simulink model "IEEE_1547_UI_TEST"  (R2018b)
settings: Solver=ode4  StartTime=0.0  StopTime=inf  FixedStep=Ts  RelTol=1e-3  EnableMultiTasking=on
PostLoadFcn:
  | Ts=40e-6; ARTEMIS_DISABLE_RTLAB_COMPATIBILTY_CHECK=1;
InitFcn:
  | Ts=40e-6; ARTEMIS_DISABLE_RTLAB_COMPATIBILTY_CHECK=1;
undefined symbols (not defined in the file or in its folder): another_event_name, I, Left, my_event_name, Right, type, V
libraries: simulink x72, powerlib_meascontrol x70, powerlib x66, artemis x4, rtlab x3, rtio_opalrt_ml605ex1 x3
(part 2 of 3)

== system IEEE_1547_UI_TEST/SC_InputsandOutputs/Subsystem9/Subsystem6 ==
  Inverter Measurements : Inport
  Bus Selector : BusSelector  OutputSignals=Inv VLL,Inv I,Inv Ptot pu,Inv Qtot pu,Inv Freq,Inv Pgen,Inv QFactor,Inv Ptot,Inv Qtot
  To Workspace : ToWorkspace  VariableName=Inv_VLL  SaveFormat=Timeseries  SampleTime=-1
  To Workspace1 : ToWorkspace  VariableName=Inv_I  SaveFormat=Timeseries  SampleTime=-1
  To Workspace2 : ToWorkspace  VariableName=Inv_Ptot_pu  SaveFormat=Timeseries  SampleTime=-1
  To Workspace3 : ToWorkspace  VariableName=Inv_Qtot_pu  SaveFormat=Timeseries  SampleTime=-1
  To Workspace4 : ToWorkspace  VariableName=Inv_Freq  SaveFormat=Timeseries  SampleTime=-1
  To Workspace5 : ToWorkspace  VariableName=Inv_Pgen  SaveFormat=Timeseries  SampleTime=-1
  To Workspace6 : ToWorkspace  VariableName=Inv_QFactor  SaveFormat=Timeseries  SampleTime=-1
  To Workspace7 : ToWorkspace  VariableName=Inv_Ptot  SaveFormat=Timeseries  SampleTime=-1
  To Workspace8 : ToWorkspace  VariableName=Inv_Qtot  SaveFormat=Timeseries  SampleTime=-1
  wires:
  Inverter Measurements/1 -> Bus Selector/1
  Bus Selector/1 -> To Workspace/1  "<Inv VLL>"
  Bus Selector/2 -> To Workspace1/1  "<Inv I>"
  Bus Selector/3 -> To Workspace2/1  "<Inv Ptot pu>"
  Bus Selector/4 -> To Workspace3/1  "<Inv Qtot pu>"
  Bus Selector/5 -> To Workspace4/1  "<Inv Freq>"
  Bus Selector/6 -> To Workspace5/1  "<Inv Pgen>"
  Bus Selector/7 -> To Workspace6/1  "<Inv QFactor>"
  Bus Selector/8 -> To Workspace7/1  "<Inv Ptot>"
  Bus Selector/9 -> To Workspace8/1  "<Inv Qtot>"

== system IEEE_1547_UI_TEST/SC_InputsandOutputs/Subsystem9/Subsystem7 ==
  Load Measurements : Inport
  Bus Selector : BusSelector  OutputSignals=Load Vph,Load Vll,Load I,Load Ppu,Load Qpu,Load PF,IR,IL,IC,PR pu,PL pu,QL pu,QC pu
  To Workspace1 : ToWorkspace  VariableName=Load_VLL  SaveFormat=Timeseries  SampleTime=-1
  To Workspace10 : ToWorkspace  VariableName=QL_pu  SaveFormat=Timeseries  SampleTime=-1
  To Workspace11 : ToWorkspace  VariableName=PL_pu  SaveFormat=Timeseries  SampleTime=-1
  To Workspace12 : ToWorkspace  VariableName=I_Capacitor  SaveFormat=Timeseries  SampleTime=-1
  To Workspace13 : ToWorkspace  VariableName=QC_PU  SaveFormat=Timeseries  SampleTime=-1
  To Workspace2 : ToWorkspace  VariableName=Load_Ptot_pu  SaveFormat=Timeseries  SampleTime=-1
  To Workspace3 : ToWorkspace  VariableName=Load_I  SaveFormat=Timeseries  SampleTime=-1
  To Workspace4 : ToWorkspace  VariableName=Load_PF  SaveFormat=Timeseries  SampleTime=-1
  To Workspace5 : ToWorkspace  VariableName=I_Inductor  SaveFormat=Timeseries  SampleTime=-1
  To Workspace6 : ToWorkspace  VariableName=I_Resistor  SaveFormat=Timeseries  SampleTime=-1
  To Workspace7 : ToWorkspace  VariableName=Load_Vph  SaveFormat=Timeseries  SampleTime=-1
  To Workspace8 : ToWorkspace  VariableName=Load_Qtot_pu  SaveFormat=Timeseries  SampleTime=-1
  To Workspace9 : ToWorkspace  VariableName=PR_pu  SaveFormat=Timeseries  SampleTime=-1
  wires:
  Load Measurements/1 -> Bus Selector/1
  Bus Selector/1 -> To Workspace7/1  "<Load Vph>"
  Bus Selector/2 -> To Workspace1/1  "<Load Vll>"
  Bus Selector/3 -> To Workspace3/1  "<Load I>"
  Bus Selector/4 -> To Workspace2/1  "<Load Ppu>"
  Bus Selector/5 -> To Workspace8/1  "<Load Qpu>"
  Bus Selector/6 -> To Workspace4/1  "<Load PF>"
  Bus Selector/7 -> To Workspace6/1  "<IR>"
  Bus Selector/8 -> To Workspace5/1  "<IL>"
  Bus Selector/9 -> To Workspace12/1  "<IC>"
  Bus Selector/10 -> To Workspace9/1  "<PR pu>"
  Bus Selector/11 -> To Workspace11/1  "<PL pu>"
  Bus Selector/12 -> To Workspace10/1  "<QL pu>"
  Bus Selector/13 -> To Workspace13/1  "<QC pu>"

== system IEEE_1547_UI_TEST/SC_InputsandOutputs/Subsystem9/Subsystem8 ==
  RLC Display Values : Inport
  Bus Selector : BusSelector  OutputSignals=Resistor (ohms),Rint (ohms),Inductor (mH),Capacitor (uF)
  To Workspace1 : ToWorkspace  VariableName=ohms_in_Rint  SaveFormat=Timeseries  SampleTime=-1
  To Workspace10 : ToWorkspace  VariableName=ohms_in_R  SaveFormat=Timeseries  SampleTime=-1
  To Workspace2 : ToWorkspace  VariableName=uF_in_C  SaveFormat=Timeseries  SampleTime=-1
  To Workspace3 : ToWorkspace  VariableName=mH_in_L  SaveFormat=Timeseries  SampleTime=-1
  wires:
  RLC Display Values/1 -> Bus Selector/1
  Bus Selector/1 -> To Workspace10/1  "<Resistor (ohms)>"
  Bus Selector/2 -> To Workspace1/1  "<Rint (ohms)>"
  Bus Selector/3 -> To Workspace3/1  "<Inductor (mH)>"
  Bus Selector/4 -> To Workspace2/1  "<Capacitor (uF)>"

== system IEEE_1547_UI_TEST/SM_SystemDynamics/ 3Phase Y Load with N/   C Bank ==
  note: Compensator for fixed time steps of 40e-6
  uC. : Inport
  AVG( RMS )1 : Subsystem
      mask Display: color('blue');disp('RMS\nAVG')
  Add1 : Sum  Inputs=2
  C1 : Subsystem
  C2 : Subsystem
  C3 : Subsystem
  Divide : Product
  Mux : Mux  Inputs=3
  Mux1 : Mux  Inputs=3
  Opposite of P_L : Constant  Value=-1
  Power per Element : Subsystem
      mask Display:
      | color('red')
      | disp('Power          \nper               \nElement       ')
  "Power, 3Ph (  Fund. Frecu. )" : Subsystem
  A : PMIOPort  Side=Left
  B : PMIOPort  Port=2  Side=Left
  C : PMIOPort  Port=3  Side=Left
  a : PMIOPort  Port=4  Side=Right
  b : PMIOPort  Port=5  Side=Right
  c : PMIOPort  Port=6  Side=Right
  P_VC : Outport
  Q_C : Outport  Port=2
  tag scope: I_C=global, P_C=global
  wires:
  uC./1 -> C1/1(uC), C3/1(uC), C2/1(uC)
  "Power, 3Ph (  Fund. Frecu. )"/2(Q) -> Q_C/1
  "Power, 3Ph (  Fund. Frecu. )"/1(P) -> [P_C]
  C2/1(V_C) -> Mux/3
  C3/2(I_C) -> Mux1/1
  C1/2(I_C) -> Mux1/2
  C3/1(V_C) -> Mux/1
  C1/1(V_C) -> Mux/2
  C2/2(I_C) -> Mux1/3
  Add1/1 -> P_VC/1
  [P_C] -> Divide/1, Add1/1
  Divide/1 -> Add1/2
  Opposite of P_L/1 -> Divide/2
  AVG( RMS )1/1(Out1) -> [I_C]
  Mux/1 -> Power per Element/1(Vabc), "Power, 3Ph (  Fund. Frecu. )"/1(Vabc)
  Mux1/1 -> Power per Element/2(Iabc), "Power, 3Ph (  Fund. Frecu. )"/2(Iabc), AVG( RMS )1/1(In1)
  connections:
  C3/RConn2 -- a/RConn1
  C1/RConn1 -- B/RConn1
  C3/RConn1 -- A/RConn1
  C2/RConn2 -- c/RConn1
  C1/RConn2 -- b/RConn1
  C2/RConn1 -- C/RConn1

== system IEEE_1547_UI_TEST/SM_SystemDynamics/ 3Phase Y Load with N/   R Bank1 ==
  ohms : Inport
  "3Ph ( P.U. ) Power, Fund. Frec." : Subsystem
  AVG( RMS )4 : Subsystem
      mask Display: color('blue');disp('RMS\nAVG')
  Mux : Mux  Inputs=3
  Mux1 : Mux  Inputs=3
  Power per Element : Subsystem
      mask Display:
      | color('red')
      | disp('Power          \nper               \nElement       ')
  R1 : Subsystem
  R2 : Subsystem
  R3 : Subsystem
  A : PMIOPort  Side=Left
  B : PMIOPort  Port=2  Side=Left
  C : PMIOPort  Port=3  Side=Left
  a : PMIOPort  Port=4  Side=Right
  b : PMIOPort  Port=5  Side=Right
  c : PMIOPort  Port=6  Side=Right
  P_RL : Outport
  Q_RL : Outport  Port=2
  tag scope: I_R=global
  wires:
  R1/1(V) -> Mux/1
  R2/2(I) -> Mux1/2
  R3/2(I) -> Mux1/3
  R1/2(I) -> Mux1/1
  R2/1(V) -> Mux/2
  R3/1(V) -> Mux/3
  "3Ph ( P.U. ) Power, Fund. Frec."/1(P) -> P_RL/1
  "3Ph ( P.U. ) Power, Fund. Frec."/2(Q) -> Q_RL/1
  ohms/1 -> R1/1(ohms), R3/1(ohms), R2/1(ohms)
  AVG( RMS )4/1(Out1) -> [I_R]
  Mux1/1 -> AVG( RMS )4/1(In1), Power per Element/2(Iabc), "3Ph ( P.U. ) Power, Fund. Frec."/2(Iabc)
  Mux/1 -> Power per Element/1(Vabc), "3Ph ( P.U. ) Power, Fund. Frec."/1(Vabc)
  connections:
  R2/RConn2 -- b/RConn1
  R3/RConn2 -- c/RConn1
  R1/RConn2 -- a/RConn1
  R1/RConn1 -- A/RConn1
  R2/RConn1 -- B/RConn1
  R3/RConn1 -- C/RConn1

== system IEEE_1547_UI_TEST/SM_SystemDynamics/ 3Phase Y Load with N/( Rint + L ) Bank ==
  mH : Inport
  Rint : Inport  Port=2
  AVG( RMS )1 : Subsystem
      mask Display: color('blue');disp('RMS\nAVG')
  Add : Sum  Inputs=2
  L1 : Subsystem
  L2 : Subsystem
  L3 : Subsystem
  Mean2 : powerlib_meascontrol/Measurements/Mean  Freq=30  Vinit=0  Ts=Ts
      settings: SourceProductName=Simscape Electrical
  Mux2 : Mux  Inputs=3
  Mux3 : Mux  Inputs=3
  Power per Element : Subsystem
      mask Display:
      | color('red')
      | disp('Power          \nper               \nElement       ')
  "Power, 3Ph (  Fund. Frecu. )" : Subsystem
  A : PMIOPort  Side=Left
  B : PMIOPort  Port=2  Side=Left
  C : PMIOPort  Port=3  Side=Left
  a : PMIOPort  Port=4  Side=Right
  b : PMIOPort  Port=5  Side=Right
  c : PMIOPort  Port=6  Side=Right
  P_L : Outport
  Q_L : Outport  Port=2
  tag scope: I_L=global
  wires:
  L1/2(I_L) -> Mux3/1
  L2/2(I_L) -> Mux3/2
  L3/2(I_L) -> Mux3/3
  mH/1 -> L3/1(mH), L2/1(mH), L1/1(mH)
  Rint/1 -> L3/2(Rint), L2/2(Rint), L1/2(Rint)
  L2/1(V_L) -> Mux2/2
  L3/1(V_L) -> Mux2/3
  "Power, 3Ph (  Fund. Frecu. )"/2(Q) -> Q_L/1
  L1/1(V_L) -> Mux2/1
  [P_C] -> Add/1
  "Power, 3Ph (  Fund. Frecu. )"/1(P) -> Add/2
  Add/1 -> Mean2/1
  AVG( RMS )1/1(Out1) -> [I_L]
  Mean2/1 -> P_L/1
  Mux2/1 -> Power per Element/1(Vabc), "Power, 3Ph (  Fund. Frecu. )"/1(Vabc)
  Mux3/1 -> Power per Element/2(Iabc), AVG( RMS )1/1(In1), "Power, 3Ph (  Fund. Frecu. )"/2(Iabc)
  connections:
  L1/RConn2 -- a/RConn1
  L2/RConn2 -- b/RConn1
  L3/RConn2 -- c/RConn1
  L3/RConn1 -- C/RConn1
  L1/RConn1 -- A/RConn1
  L2/RConn1 -- B/RConn1

== system IEEE_1547_UI_TEST/SM_SystemDynamics/Inverter Measurements/AVG( RMS )2 ==
  In1 : Inport
  Mean : powerlib_meascontrol/Measurements/Mean  Freq=60  Vinit=0  Ts=0
      settings: SourceProductName=Simscape Electrical
  RMS : powerlib_meascontrol/Measurements/RMS  TrueRMS=on  Freq=60  RMSInit=120  Ts=Ts
      settings: SourceProductName=Simscape Electrical
  Out1 : Outport
  wires:
  Mean/1 -> Out1/1
  RMS/1 -> Mean/1
  In1/1 -> RMS/1

== system IEEE_1547_UI_TEST/SM_SystemDynamics/Inverter Measurements/AVG( RMS )6 ==
  In1 : Inport
  Mean : powerlib_meascontrol/Measurements/Mean  Freq=60  Vinit=0  Ts=Ts
      settings: SourceProductName=Simscape Electrical
  RMS : powerlib_meascontrol/Measurements/RMS  TrueRMS=on  Freq=60  RMSInit=120  Ts=Ts
      settings: SourceProductName=Simscape Electrical
  Out1 : Outport
  wires:
  Mean/1 -> Out1/1
  RMS/1 -> Mean/1
  In1/1 -> RMS/1

== system IEEE_1547_UI_TEST/SM_SystemDynamics/Inverter Measurements/Inverter Performance ==
  P_inv_pu : Inport
  P_Load_pu : Inport  Port=2
  Q_inv_pu : Inport  Port=3
  Q_L_pu : Inport  Port=4
  Q_C_pu : Inport  Port=5
  Abs : Abs
  Abs1 : Abs
  Add : Sum
  Add1 : Sum
  Compare To Constant1 : simulink/Logic and Bit Operations/Compare To Constant  relop=<  const=0  OutDataTypeStr=boolean
  Compare To Constant3 : simulink/Logic and Bit Operations/Compare To Constant  relop=>  const=0  OutDataTypeStr=boolean
  Divide : Product  Inputs=*/  SaturateOnIntegerOverflow=on  RndMeth=Zero
  Divide1 : Product  Inputs=**  SaturateOnIntegerOverflow=on  RndMeth=Zero
  Divide2 : Product  Inputs=**  SaturateOnIntegerOverflow=on  RndMeth=Zero
  Divide3 : Product  Inputs=**  SaturateOnIntegerOverflow=on  RndMeth=Zero
  Divide4 : Product  Inputs=/*  SaturateOnIntegerOverflow=on  RndMeth=Zero
  Divide5 : Product  Inputs=*/  SaturateOnIntegerOverflow=on  RndMeth=Zero
  Divide6 : Product  Commented=on  Inputs=**  SaturateOnIntegerOverflow=on  RndMeth=Zero
  Divide8 : Product  Commented=on  Inputs=**  SaturateOnIntegerOverflow=on  RndMeth=Zero
  Saturation : Saturate  Commented=through  UpperLimit=inf  LowerLimit=0.0001
  Saturation1 : Saturate  Commented=through  UpperLimit=inf  LowerLimit=0.0001
  Sqrt : Sqrt  SaturateOnIntegerOverflow=on
  Sqrt1 : Sqrt  Commented=on  SaturateOnIntegerOverflow=on
  Sqrt2 : Sqrt  Commented=on  SaturateOnIntegerOverflow=on
  P Gen : Outport
  Q factor : Outport  Port=2
  wires:
  P_inv_pu/1 -> Divide/1
  Compare To Constant3/1 -> Divide1/1
  Compare To Constant1/1 -> Divide2/2
  Q_inv_pu/1 -> Compare To Constant1/1, Compare To Constant3/1, Abs/1
  Divide1/1 -> Add/2
  Abs/1 -> Divide1/2, Divide2/1
  Q_L_pu/1 -> Add/1
  Divide2/1 -> Add1/1
  Q_C_pu/1 -> Abs1/1
  Add/1 -> Divide3/1, Divide5/1
  Divide3/1 -> Sqrt/1
  Sqrt/1 -> Divide4/2
  Divide4/1 -> Q factor/1
  Abs1/1 -> Add1/2
  Divide5/1 -> Sqrt1/1
  Sqrt1/1 -> Divide6/1
  Divide6/1 -> ?  "Freq_Island"
  ? -> Divide6/2  "Freq_EPS"
  Divide/1 -> Sqrt2/1, P Gen/1
  Sqrt2/1 -> Divide8/2
  ? -> Divide8/1  "Vph_Uti"
  Divide8/1 -> ?  "V_Island"
  P_Load_pu/1 -> Saturation1/1
  Add1/1 -> Saturation/1, Divide3/2
  Saturation/1 -> Divide5/2
  Saturation1/1 -> Divide/2, Divide4/1

== system IEEE_1547_UI_TEST/SM_SystemDynamics/Inverter Measurements/Phase Angle Meter1 ==
  Vabc : Inport
  Iabc : Inport  Port=2
  Constant : Constant  Value=-1
  Cos : Trigonometry  Operator=cos
  Gain : Gain  Gain=pi/180
  PLL (3ph) : powerlib_meascontrol/PLL/PLL (3ph)  Fmin=30  Par_Init=[0, 60]  ParK=[180, 3200, 1]  TcD=1e-4  MaxRateChangeFreq=12  FilterCutOffFreq=25  Ts=Ts  AGC=on
  Positive-Sequence (PLL-Driven) : powerlib_meascontrol/Measurements/Positive-Sequence (PLL-Driven)  Finit=60  Fmin=45  InInit=[1, 0]  Ts=Ts
      settings: SourceProductName=Simscape Power Systems  SourceProductBaseCode=PS
  Product : Product  Inputs=3
  Sign : Signum
  Θ : Outport
  pf : Outport  Port=2
  wires:
  PLL (3ph)/1 -> Positive-Sequence (PLL-Driven)/1
  PLL (3ph)/2 -> Positive-Sequence (PLL-Driven)/2
  Iabc/1 -> Positive-Sequence (PLL-Driven)/3
  Vabc/1 -> PLL (3ph)/1
  Positive-Sequence (PLL-Driven)/2 -> Gain/1, Sign/1, Θ/1
  Product/1 -> pf/1
  Gain/1 -> Cos/1
  Cos/1 -> Product/3
  Constant/1 -> Product/2
  Sign/1 -> Product/1

== system IEEE_1547_UI_TEST/SM_SystemDynamics/Inverter Measurements/Power, 3Ph ( Fundamental Frecuency ) ==
  note: Per Unit Converter
  note: Per Unit Converter
  Vabc : Inport
  Iabc : Inport  Port=2
  Inv Size : Inport  Port=3
  Divide : Product  Inputs=*/
  Divide1 : Product  Inputs=*/
  Gain : Gain
  Gain1 : Gain
  Mean1 : powerlib_meascontrol/Measurements/Mean  Freq=30  Vinit=0  Ts=Ts
      settings: SourceProductName=Simscape Electrical
  Mean2 : powerlib_meascontrol/Measurements/Mean  Freq=30  Vinit=0  Ts=Ts
      settings: SourceProductName=Simscape Electrical
  PLL (3ph) : powerlib_meascontrol/PLL/PLL (3ph)  Fmin=45  Par_Init=[0, 60]  ParK=[180, 3200, 1]  TcD=1e-4  MaxRateChangeFreq=12  FilterCutOffFreq=25  Ts=Ts  AGC=on
      settings: SourceProductName=Simscape Electrical
  Power ( Fundamental Frecuency ) : powerlib_meascontrol/Measurements/Power (PLL-Driven, Positive-Sequence)  Finit=60  Fmin=45  Vinit=[1, 0]  Iinit=[1, 0]  Ts=Ts
      settings: SourceProductName=Simscape Electrical  SourceProductBaseCode=PS
  P : Outport
  Ppu : Outport  Port=2
  Q : Outport  Port=3
  Qpu : Outport  Port=4
  Inv Freq : Outport  Port=5
  wires:
  Mean2/1 -> P/1, Divide/1
  Gain/1 -> Divide/2
  Power ( Fundamental Frecuency )/1 -> Mean2/1
  Mean1/1 -> Q/1, Divide1/1
  Gain1/1 -> Divide1/2
  Power ( Fundamental Frecuency )/2 -> Mean1/1
  Divide/1 -> Ppu/1
  Divide1/1 -> Qpu/1
  Inv Size/1 -> Gain/1, Gain1/1
  PLL (3ph)/1 -> Inv Freq/1, Power ( Fundamental Frecuency )/1
  PLL (3ph)/2 -> Power ( Fundamental Frecuency )/2
  Vabc/1 -> Power ( Fundamental Frecuency )/3, PLL (3ph)/1
  Iabc/1 -> Power ( Fundamental Frecuency )/4

== system IEEE_1547_UI_TEST/SM_SystemDynamics/MASTER CONTROL OUTPUTS/INVERTER MEASURES ==
  Bus Creator : BusCreator  Inputs=10
  Inv Freq : Gain
  Inv I : Gain
  Inv Pgen : Gain
  Inv Ptot : Gain
  Inv Ptot pu : Gain
  Inv Qfactor : Gain
  Inv Qtot : Gain
  Inv Qtot pu : Gain
  Inv Vph : Gain
  Inv Vph pu : Gain  Gain=1/277
  Subsystem : Subsystem
  Subsystem1 : Subsystem
  Inverter Measures : Outport
  wires:
  Subsystem/1(Out1) -> Inv Vph pu/1, Inv Vph/1  "Inv Vph"
  [Pinv_pu] -> Inv Ptot pu/1  "Inv Ptot pu"
  [Qinv_pu] -> Inv Qtot pu/1  "Inv Qtot pu"
  Subsystem1/1(Out1) -> Inv Freq/1  "Inv Freq"
  [p_gen] -> Inv Pgen/1  "Inv Pgen"
  [q_Factor] -> Inv Qfactor/1  "Inv QFactor"
  [P_inv] -> Inv Ptot/1  "Inv Ptot"
  [Q_inv] -> Inv Qtot/1  "Inv Qtot"
  [inv_I] -> Inv I/1  "Inv I"
  Bus Creator/1 -> Inverter Measures/1
  Inv I/1 -> Bus Creator/3  "Inv I"
  Inv Freq/1 -> Bus Creator/6  "Inv Freq"
  Inv Pgen/1 -> Bus Creator/7  "Inv Pgen"
  Inv Ptot/1 -> Bus Creator/9  "Inv Ptot"
  Inv Ptot pu/1 -> Bus Creator/4  "Inv Ptot pu"
  Inv Qfactor/1 -> Bus Creator/8  "Inv QFactor"
  Inv Qtot/1 -> Bus Creator/10  "Inv Qtot"
  Inv Qtot pu/1 -> Bus Creator/5  "Inv Qtot pu"
  Inv Vph/1 -> Bus Creator/1  "Inv Vph"
  Inv Vph pu/1 -> Bus Creator/2  "Inv Vph PU"
  [stop_ametek] -> Subsystem/1(trig)
  [inv_Vph] -> Subsystem/2(input)  "Inv Vph"
  [stop_ametek] -> Subsystem1/1(trig)
  [Inv_Freq] -> Subsystem1/2(input)  "Inv Freq"

== system IEEE_1547_UI_TEST/SM_SystemDynamics/MASTER CONTROL OUTPUTS/LOAD MEASURES ==
  Bus Creator : BusCreator  Inputs=15
  IC : Gain
  IL : Gain
  IR : Gain
  Load I : Gain
  Load PF : Gain
  Load Ppu : Gain
  Load Qpu : Gain
  Load Vph : Gain
  Load Vph pu : Gain  Gain=1/277
  PL pu : Gain
  PLoad Watts : Gain
  PR pu : Gain
  QC pu : Gain
  QL pu : Gain
  QLoad Vars : Gain
  Load Measures : Outport
  wires:
  [pf] -> Load PF/1  "Load PF"
  [load_Vph] -> Load Vph pu/1, Load Vph/1  "Load Vph"
  [load_I] -> Load I/1  "Load I"
  [PLpu] -> Load Ppu/1  "Load Ppu"
  [QLpu] -> Load Qpu/1  "Load Qpu"
  [I_R] -> IR/1  "IR"
  [I_L] -> IL/1  "IL"
  [I_C] -> IC/1  "IC"
  [P_RL] -> PR pu/1  "PR pu"
  [P_L] -> PL pu/1  "PL pu"
  [Q_L] -> QL pu/1  "QL pu"
  [Q_C] -> QC pu/1  "QC pu"
  Bus Creator/1 -> Load Measures/1
  Load Vph/1 -> Bus Creator/1  "Load Vph"
  Load Vph pu/1 -> Bus Creator/2  "Load Vph pu"
  Load I/1 -> Bus Creator/3  "Load I"
  Load Ppu/1 -> Bus Creator/4  "Load Ppu"
  Load Qpu/1 -> Bus Creator/5  "Load Qpu"
  Load PF/1 -> Bus Creator/6  "Load PF"
  IR/1 -> Bus Creator/7  "IR"
  IL/1 -> Bus Creator/8  "IL"
  IC/1 -> Bus Creator/9  "IC"
  PR pu/1 -> Bus Creator/10  "PR pu"
  PL pu/1 -> Bus Creator/11  "PL pu"
  QL pu/1 -> Bus Creator/12  "QL pu"
  QC pu/1 -> Bus Creator/13  "QC pu"
  QLoad Vars/1 -> Bus Creator/15  "QLoad Vars"
  PLoad Watts/1 -> Bus Creator/14  "PLoad Watts"
  [P_load_Watts] -> PLoad Watts/1
  [Q_load_Vars] -> QLoad Vars/1

== system IEEE_1547_UI_TEST/SM_SystemDynamics/MASTER CONTROL OUTPUTS/RLC DISPLAYED VALUES ==
  Bus Creator : BusCreator  Inputs=7
  C in uF : Gain
  FreqPCC : Gain
  L in mh : Gain
  R in ohms : Gain
  Rint in ohms : Gain
  Spare O1 : Gain
  Spare O2 : Gain
  RLC Displayed Values : Outport
  wires:
  [ohms7] -> Rint in ohms/1
  [ohms2] -> R in ohms/1
  [uF2] -> C in uF/1
  [mH2] -> L in mh/1
  Bus Creator/1 -> RLC Displayed Values/1
  C in uF/1 -> Bus Creator/4  "Capacitor (uF)"
  R in ohms/1 -> Bus Creator/1  "Resistor (ohms)"
  Rint in ohms/1 -> Bus Creator/2  "Rint (ohms)"
  L in mh/1 -> Bus Creator/3  "Inductor (mH)"
  FreqPCC/1 -> Bus Creator/5  "Freq PCC"
  [FreqPCC] -> FreqPCC/1
  Spare O2/1 -> Bus Creator/6  "Spare O2"
  [Spare_O2] -> Spare O2/1
  Spare O1/1 -> Bus Creator/7  "Spare O1"
  [Spare_O1] -> Spare O1/1

== system IEEE_1547_UI_TEST/SM_SystemDynamics/MASTER CONTROL OUTPUTS/SPARE MEASURES ==
  Bus Creator2 : BusCreator  Inputs=5
  Islanding Signal : Gain  Gain=-1
  OpMonitor : rtlab/Monitoring/OpMonitor  compute_time=off  real_step=off  idle_time=off  nb_overruns=on  user_time=off  user_name=my_event_name,another_event_name
      settings: SourceProductName=RT-LAB
  Phase Angle : Gain
  Spare O3 : Gain
  pf_inv : Gain
  Spare Measures : Outport
  wires:
  [Islanding_Test] -> Islanding Signal/1
  [pf_inv] -> pf_inv/1
  [Spare_O3] -> Spare O3/1
  [Phase_Angle] -> Phase Angle/1
  Bus Creator2/1 -> Spare Measures/1
  Islanding Signal/1 -> Bus Creator2/3  "Island Sig"
  Phase Angle/1 -> Bus Creator2/2  "Phase Angle"
  Spare O3/1 -> Bus Creator2/5  "Spare O3"
  pf_inv/1 -> Bus Creator2/1  "pf_inv"
  OpMonitor/1 -> Bus Creator2/4  "Overruns"

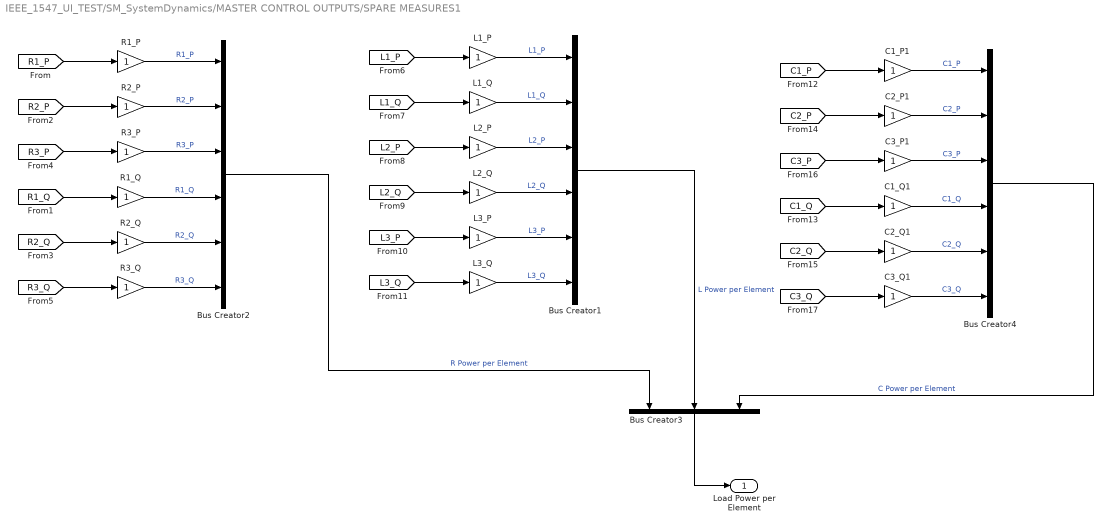
== system IEEE_1547_UI_TEST/SM_SystemDynamics/MASTER CONTROL OUTPUTS/SPARE MEASURES1 ==
  Bus Creator1 : BusCreator  Inputs=6
  Bus Creator2 : BusCreator  Inputs=6
  Bus Creator3 : BusCreator  Inputs=3
  Bus Creator4 : BusCreator  Inputs=6
  C1_P1 : Gain
  C1_Q1 : Gain
  C2_P1 : Gain
  C2_Q1 : Gain
  C3_P1 : Gain
  C3_Q1 : Gain
  L1_P : Gain
  L1_Q : Gain
  L2_P : Gain
  L2_Q : Gain
  L3_P : Gain
  L3_Q : Gain
  R1_P : Gain
  R1_Q : Gain
  R2_P : Gain
  R2_Q : Gain
  R3_P : Gain
  R3_Q : Gain
  Load Power per Element : Outport
  wires:
  R3_P/1 -> Bus Creator2/3  "R3_P"
  R2_P/1 -> Bus Creator2/2  "R2_P"
  R2_Q/1 -> Bus Creator2/5  "R2_Q"
  R1_P/1 -> Bus Creator2/1  "R1_P"
  R1_Q/1 -> Bus Creator2/4  "R1_Q"
  R3_Q/1 -> Bus Creator2/6  "R3_Q"
  [R1_P] -> R1_P/1
  [R1_Q] -> R1_Q/1
  [R2_P] -> R2_P/1
  [R3_P] -> R3_P/1
  [R2_Q] -> R2_Q/1
  [R3_Q] -> R3_Q/1
  Bus Creator1/1 -> Bus Creator3/2  "L Power per Element"
  L2_P/1 -> Bus Creator1/3  "L2_P"
  [L3_P] -> L3_P/1
  L3_P/1 -> Bus Creator1/5  "L3_P"
  [L3_Q] -> L3_Q/1
  [L1_Q] -> L1_Q/1
  [L1_P] -> L1_P/1
  L2_Q/1 -> Bus Creator1/4  "L2_Q"
  [L2_Q] -> L2_Q/1
  L1_P/1 -> Bus Creator1/1  "L1_P"
  L1_Q/1 -> Bus Creator1/2  "L1_Q"
  L3_Q/1 -> Bus Creator1/6  "L3_Q"
  [L2_P] -> L2_P/1
  Bus Creator3/1 -> Load Power per Element/1
  Bus Creator2/1 -> Bus Creator3/1  "R Power per Element"
  C2_P1/1 -> Bus Creator4/2  "C2_P"
  [C3_P] -> C3_P1/1
  C3_P1/1 -> Bus Creator4/3  "C3_P"
  [C3_Q] -> C3_Q1/1
  [C1_Q] -> C1_Q1/1
  [C1_P] -> C1_P1/1
  C2_Q1/1 -> Bus Creator4/5  "C2_Q"
  [C2_Q] -> C2_Q1/1
  C1_P1/1 -> Bus Creator4/1  "C1_P"
  C1_Q1/1 -> Bus Creator4/4  "C1_Q"
  C3_Q1/1 -> Bus Creator4/6  "C3_Q"
  [C2_P] -> C2_P1/1
  Bus Creator4/1 -> Bus Creator3/3  "C Power per Element"

== system IEEE_1547_UI_TEST/SM_SystemDynamics/MASTER CONTROL OUTPUTS/SPARE MEASURES2 ==
  Bus Creator2 : BusCreator  Inputs=12
  S1_P : Gain
  S1_P_Pu : Gain
  S1_Q : Gain
  S1_Q_Pu : Gain
  S2_P : Gain
  S2_P_Pu : Gain
  S2_Q : Gain
  S2_Q_Pu : Gain
  S3_P : Gain
  S3_P_Pu : Gain
  S3_Q : Gain
  S3_Q_Pu : Gain
  Switch Power : Outport
  wires:
  S3_P/1 -> Bus Creator2/3  "S3_P_Watts"
  S2_P/1 -> Bus Creator2/2  "S2_P_Watts"
  S2_Q/1 -> Bus Creator2/5  "S2_Q_Vars"
  S1_P/1 -> Bus Creator2/1  "S1_P_Watts"
  S1_Q/1 -> Bus Creator2/4  "S1_Q_Vars"
  S3_Q/1 -> Bus Creator2/6  "S3_Q_Vars"
  [S1_Watts] -> S1_P/1
  [S1_Vars] -> S1_Q/1
  [S2_Watts] -> S2_P/1
  [S3_Watts] -> S3_P/1
  Bus Creator2/1 -> Switch Power/1  "Switch Power"
  [S3_Vars] -> S3_Q/1
  [S2_Vars] -> S2_Q/1
  [S3_P_Pu] -> S3_P_Pu/1
  [S3_Q_Pu] -> S3_Q_Pu/1
  S3_P_Pu/1 -> Bus Creator2/9  "S3_P_Pu"
  S3_Q_Pu/1 -> Bus Creator2/12  "S3_Q_Pu"
  [S1_P_Pu] -> S1_P_Pu/1
  S1_P_Pu/1 -> Bus Creator2/7  "S1_P_Pu"
  S1_Q_Pu/1 -> Bus Creator2/10  "S1_Q_Pu"
  [S1_Q_Pu] -> S1_Q_Pu/1
  [S2_P_Pu] -> S2_P_Pu/1
  S2_P_Pu/1 -> Bus Creator2/8  "S2_P_Pu"
  [S2_Q_Pu] -> S2_Q_Pu/1
  S2_Q_Pu/1 -> Bus Creator2/11  "S2_Q_Pu"

== system IEEE_1547_UI_TEST/SM_SystemDynamics/MASTER CONTROL OUTPUTS/UTILITY MEASURES ==
  Bus Creator : BusCreator  Inputs=7
  PFun : Gain
  QFun : Gain
  Uti I : Gain
  Uti Ppu : Gain
  Uti Qpu : Gain
  Uti Vph : Gain
  Uti Vph pu : Gain  Gain=1/277
  Utility Measures : Outport
  wires:
  Bus Creator/1 -> Utility Measures/1
  [uti_I] -> Uti I/1  "Utility I"
  [Vph_Uti] -> Uti Vph pu/1, Uti Vph/1  "Utility Vph"
  [Puti_pu] -> Uti Ppu/1  "Utility Ppu"
  [Quti_pu] -> Uti Qpu/1  "Utility Qpu"
  [Puti_Watts] -> PFun/1
  [Quti_Vars] -> QFun/1
  Uti I/1 -> Bus Creator/3  "Utility I"
  Uti Vph/1 -> Bus Creator/1  "Utility Vph"
  Uti Qpu/1 -> Bus Creator/5  "Utility Qpu"
  Uti Ppu/1 -> Bus Creator/4  "Utility Ppu"
  Uti Vph pu/1 -> Bus Creator/2  "Utility Vph pu"
  PFun/1 -> Bus Creator/6  "Puti_Watts"
  QFun/1 -> Bus Creator/7  "Quti_Vars"

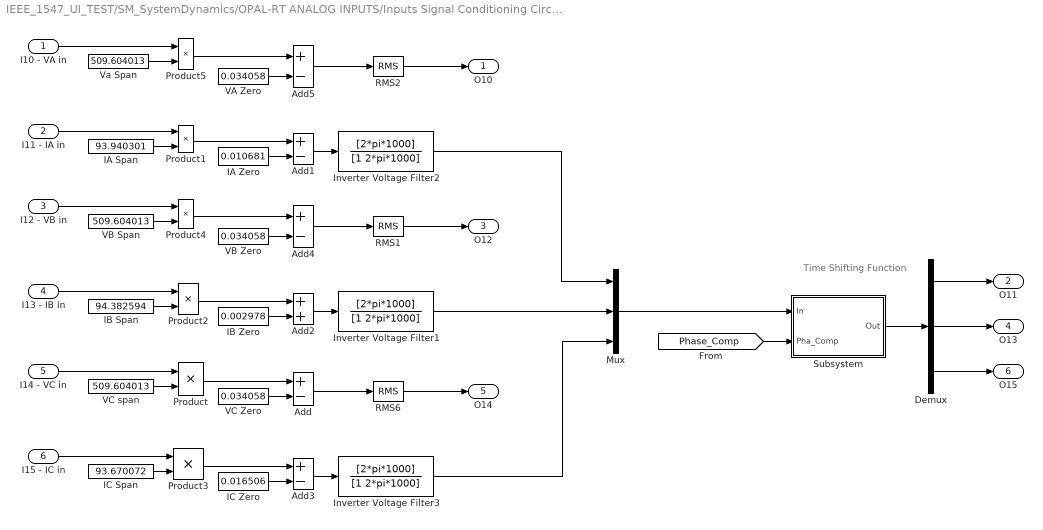
== system IEEE_1547_UI_TEST/SM_SystemDynamics/OPAL-RT ANALOG INPUTS/Inputs Signal Conditioning Circuit ==
  note: Time Shifting
      | Function
  I10 - VA in : Inport
  I11 - IA in : Inport  Port=2
  I12 - VB in : Inport  Port=3
  I13 - IB in : Inport  Port=4
  I14 - VC in : Inport  Port=5
  I15 - IC in : Inport  Port=6
  Add{,1,3..5} (5 alike) : Sum  Inputs=+-
  Add2 : Sum
  Demux : Demux  Outputs=3
  IA Span : Constant  Value=93.940301
  IA Zero : Constant  Value=0.010681
  IB Span : Constant  Value=94.382594
  IB Zero : Constant  Value=0.002978
  IC Span : Constant  Value=93.670072
  IC Zero : Constant  Value=0.016506
  Inverter Voltage Filter1 : TransferFcn  Numerator=[2*pi*1000]  Denominator=[1 2*pi*1000]
  Inverter Voltage Filter2 : TransferFcn  Numerator=[2*pi*1000]  Denominator=[1 2*pi*1000]
  Inverter Voltage Filter3 : TransferFcn  Numerator=[2*pi*1000]  Denominator=[1 2*pi*1000]
  Mux : Mux  Inputs=3
  Product{,1..5} (6 alike) : Product
  RMS1 : powerlib_meascontrol/Measurements/RMS  TrueRMS=on  Freq=60  RMSInit=120  Ts=0
      settings: SourceProductName=Simscape Electrical
  RMS2 : powerlib_meascontrol/Measurements/RMS  TrueRMS=on  Freq=60  RMSInit=120  Ts=0
      settings: SourceProductName=Simscape Electrical
  RMS6 : powerlib_meascontrol/Measurements/RMS  TrueRMS=on  Freq=60  RMSInit=120  Ts=0
      settings: SourceProductName=Simscape Electrical
  Subsystem : Subsystem
  VA Zero : Constant  Value=0.034058
  VB Span : Constant  Value=509.604013
  VB Zero : Constant  Value=0.034058
  VC Zero : Constant  Value=0.034058
  VC span : Constant  Value=509.604013
  Va Span : Constant  Value=509.604013
  "O10 " : Outport
  "O11 " : Outport  Port=2
  " O12" : Outport  Port=3
  " O13" : Outport  Port=4
  " O14" : Outport  Port=5
  " O15" : Outport  Port=6
  wires:
  RMS2/1 -> "O10 "/1
  IB Span/1 -> Product2/2
  VC span/1 -> Product/2
  IC Span/1 -> Product3/2
  VC Zero/1 -> Add/2
  Product/1 -> Add/1
  VB Span/1 -> Product4/2
  Add4/1 -> RMS1/1
  IB Zero/1 -> Add2/2
  IC Zero/1 -> Add3/2
  Product3/1 -> Add3/1
  Add1/1 -> Inverter Voltage Filter2/1
  Add2/1 -> Inverter Voltage Filter1/1
  Product2/1 -> Add2/1
  Add/1 -> RMS6/1
  IA Span/1 -> Product1/2
  Add3/1 -> Inverter Voltage Filter3/1
  Add5/1 -> RMS2/1
  Va Span/1 -> Product5/2
  I10 - VA in/1 -> Product5/1
  Inverter Voltage Filter3/1 -> Mux/3
  Inverter Voltage Filter2/1 -> Mux/1
  RMS1/1 -> " O12"/1
  I11 - IA in/1 -> Product1/1
  I12 - VB in/1 -> Product4/1
  I14 - VC in/1 -> Product/1
  I13 - IB in/1 -> Product2/1
  I15 - IC in/1 -> Product3/1
  RMS6/1 -> " O14"/1
  Inverter Voltage Filter1/1 -> Mux/2
  VB Zero/1 -> Add4/2
  Product4/1 -> Add4/1
  IA Zero/1 -> Add1/2
  Product1/1 -> Add1/1
  VA Zero/1 -> Add5/2
  Product5/1 -> Add5/1
  Mux/1 -> Subsystem/1(In)
  Subsystem/1(Out) -> Demux/1
  [Phase_Comp] -> Subsystem/2("Pha_Comp ")
  Demux/1 -> "O11 "/1
  Demux/2 -> " O13"/1
  Demux/3 -> " O15"/1

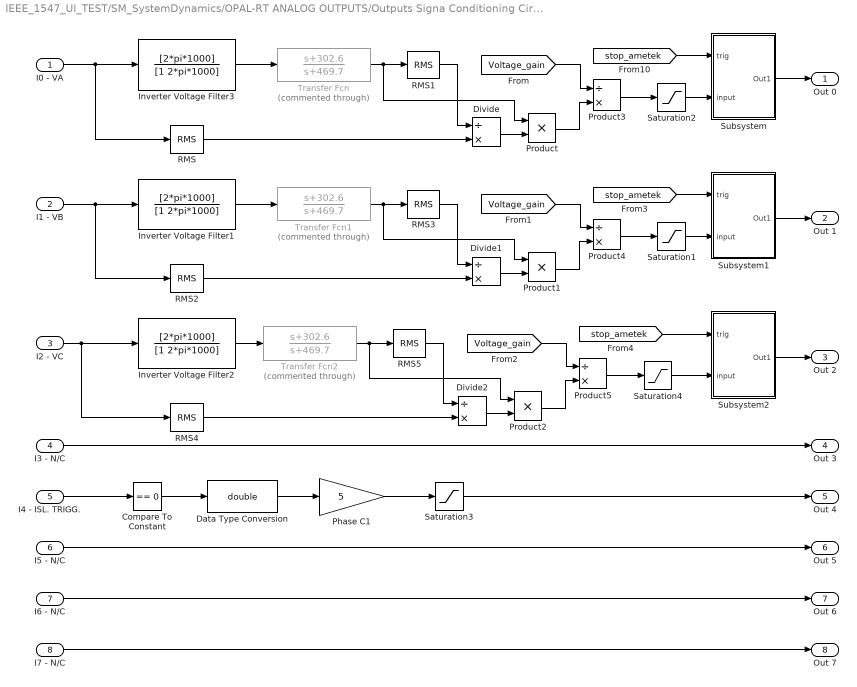
== system IEEE_1547_UI_TEST/SM_SystemDynamics/OPAL-RT ANALOG OUTPUTS/Outputs Signa Conditioning Circuit ==
  I0 - VA : Inport
  I1 - VB : Inport  Port=2
  I2 - VC : Inport  Port=3
  I3 - N/C : Inport  Port=4
  I4 - ISL. TRIGG. : Inport  Port=5
  I5 - N/C : Inport  Port=6
  I6 - N/C : Inport  Port=7
  I7 - N/C : Inport  Port=8
  Compare To Constant : simulink/Logic and Bit Operations/Compare To Constant  relop===  const=0  OutDataTypeStr=boolean
  Data Type Conversion : DataTypeConversion  OutDataTypeStr=double
  Divide : Product  Inputs=/*
  Divide1 : Product  Inputs=/*
  Divide2 : Product  Inputs=/*
  Inverter Voltage Filter1 : TransferFcn  Numerator=[2*pi*1000]  Denominator=[1 2*pi*1000]
  Inverter Voltage Filter2 : TransferFcn  Numerator=[2*pi*1000]  Denominator=[1 2*pi*1000]
  Inverter Voltage Filter3 : TransferFcn  Numerator=[2*pi*1000]  Denominator=[1 2*pi*1000]
  Phase C1 : Gain  Gain=5
  Product : Product
  Product1 : Product
  Product2 : Product
  Product3 : Product  Inputs=/*
  Product4 : Product  Inputs=/*
  Product5 : Product  Inputs=/*
  RMS{,1..5} (6 alike) : powerlib_meascontrol/Measurements/RMS  TrueRMS=on  Freq=60  RMSInit=120  Ts=Ts
      settings: SourceProductName=Simscape Electrical
  Saturation1 : Saturate  UpperLimit=10.2  LowerLimit=-10.2
  Saturation2 : Saturate  UpperLimit=10.2  LowerLimit=-10.2
  Saturation3 : Saturate  UpperLimit=5  LowerLimit=0
  Saturation4 : Saturate  UpperLimit=10.2  LowerLimit=-10.2
  Subsystem : Subsystem
  Subsystem1 : Subsystem
  Subsystem2 : Subsystem
  Transfer Fcn : TransferFcn  Commented=through  Numerator=[1 302.6]  Denominator=[1 469.7]
  Transfer Fcn1 : TransferFcn  Commented=through  Numerator=[1 302.6]  Denominator=[1 469.7]
  Transfer Fcn2 : TransferFcn  Commented=through  Numerator=[1 302.6]  Denominator=[1 469.7]
  Out 0 : Outport
  Out 1 : Outport  Port=2
  Out 2 : Outport  Port=3
  Out 3 : Outport  Port=4
  Out 4 : Outport  Port=5
  Out 5 : Outport  Port=6
  Out 6 : Outport  Port=7
  Out 7 : Outport  Port=8
  wires:
  I3 - N/C/1 -> Out 3/1
  I5 - N/C/1 -> Out 5/1
  I6 - N/C/1 -> Out 6/1
  I7 - N/C/1 -> Out 7/1
  I4 - ISL. TRIGG./1 -> Compare To Constant/1
  Saturation3/1 -> Out 4/1
  Compare To Constant/1 -> Data Type Conversion/1
  Data Type Conversion/1 -> Phase C1/1
  Inverter Voltage Filter3/1 -> Transfer Fcn/1
  I0 - VA/1 -> RMS/1, Inverter Voltage Filter3/1
  Transfer Fcn/1 -> Product/1, RMS1/1
  RMS/1 -> Divide/2
  RMS1/1 -> Divide/1
  Divide/1 -> Product/2
  Product3/1 -> Saturation2/1
  Saturation2/1 -> Subsystem/2(input)
  Phase C1/1 -> Saturation3/1
  Product/1 -> Product3/2
  [Voltage_gain] -> Product3/1
  Subsystem/1(Out1) -> Out 0/1
  [stop_ametek] -> Subsystem/1(trig)
  Product1/1 -> Product4/2
  Transfer Fcn1/1 -> Product1/1, RMS3/1
  RMS2/1 -> Divide1/2
  [Voltage_gain] -> Product4/1
  [stop_ametek] -> Subsystem1/1(trig)
  Product4/1 -> Saturation1/1
  Divide1/1 -> Product1/2
  Saturation1/1 -> Subsystem1/2(input)
  RMS3/1 -> Divide1/1
  Inverter Voltage Filter1/1 -> Transfer Fcn1/1
  I1 - VB/1 -> RMS2/1, Inverter Voltage Filter1/1
  Product2/1 -> Product5/2
  Transfer Fcn2/1 -> Product2/1, RMS5/1
  RMS4/1 -> Divide2/2
  [Voltage_gain] -> Product5/1
  [stop_ametek] -> Subsystem2/1(trig)
  Product5/1 -> Saturation4/1
  Divide2/1 -> Product2/2
  Saturation4/1 -> Subsystem2/2(input)
  RMS5/1 -> Divide2/1
  Inverter Voltage Filter2/1 -> Transfer Fcn2/1
  I2 - VC/1 -> RMS4/1, Inverter Voltage Filter2/1
  Subsystem1/1(Out1) -> Out 1/1
  Subsystem2/1(Out1) -> Out 2/1

== system IEEE_1547_UI_TEST/SM_SystemDynamics/PHIL SOFTWARE SIDE CURRENT SOURCES/Subsystem ==
  trig : Inport
  input : Inport  Port=2
  Constant : Constant  Value=0
  Switch : Switch  Criteria=u2 > Threshold
  Out1 : Outport
  wires:
  Switch/1 -> Out1/1
  trig/1 -> Switch/2
  Constant/1 -> Switch/3
  input/1 -> Switch/1

== system IEEE_1547_UI_TEST/SM_SystemDynamics/PHIL SOFTWARE SIDE CURRENT SOURCES/Subsystem1 ==
  trig : Inport
  input : Inport  Port=2
  Constant : Constant  Value=0
  Switch : Switch  Criteria=u2 > Threshold
  Out1 : Outport
  wires:
  Switch/1 -> Out1/1
  trig/1 -> Switch/2
  Constant/1 -> Switch/3
  input/1 -> Switch/1

== system IEEE_1547_UI_TEST/SM_SystemDynamics/PHIL SOFTWARE SIDE CURRENT SOURCES/Subsystem2 ==
  trig : Inport
  input : Inport  Port=2
  Constant : Constant  Value=0
  Switch : Switch  Criteria=u2 > Threshold
  Out1 : Outport
  wires:
  Switch/1 -> Out1/1
  trig/1 -> Switch/2
  Constant/1 -> Switch/3
  input/1 -> Switch/1

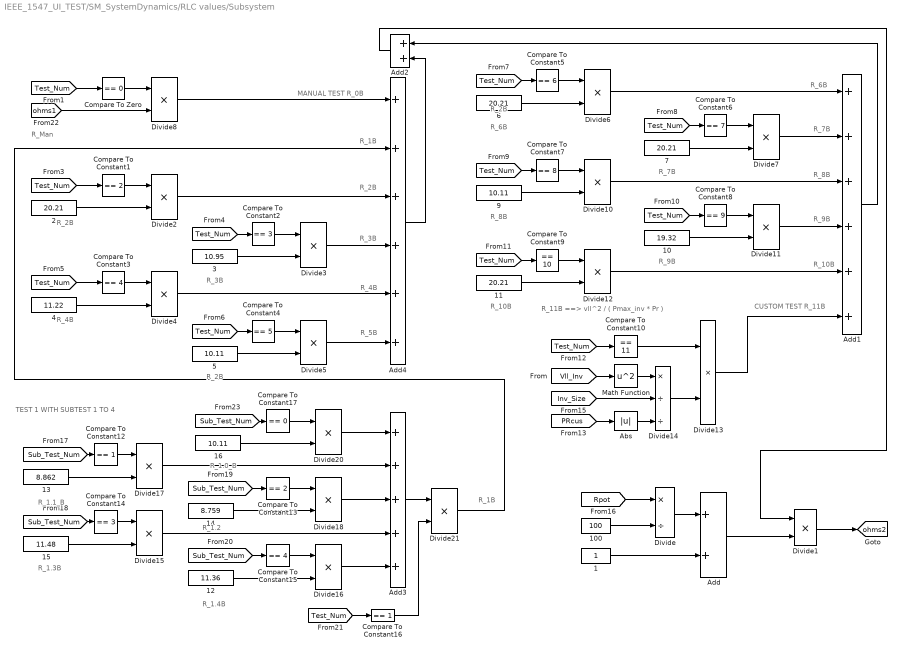
== system IEEE_1547_UI_TEST/SM_SystemDynamics/RLC values/Subsystem ==
  note: R_2B
  note: R_4B
  note: TEST 1 WITH SUBTEST 1 TO 4
  note: R_3B
  note: R_4B
  note: R_7B
  note: MANUAL TEST R_0B
  note: R_9B
  note: CUSTOM TEST R_11B
  note: R_5B
  note: R_Man
  note: R_11B ==> vll^2 / ( Pmax_inv * Pr )
  note: R_8B
  note: R_2B
  note: R_1.2
  note: R_10B
  note: R_6B
  note: R_2B
  note: R_1.3B
  note: R_10B
  note: R_9B
  note: R_8B
  note: R_1B
  note: R_1.0_B
  note: R_6B
  note: R_2B
  note: R_3B
  note: R_1.1_B
  note: R_1B
  note: R_1.4B
  note: R_7B
  1 : Constant
  10 : Constant  Value=19.32
  100 : Constant  Value=100
  {2,6..7,11} (4 alike) : Constant  Value=20.21
  12 : Constant  Value=11.36
  13 : Constant  Value=8.862
  14 : Constant  Value=8.759
  15 : Constant  Value=11.48
  16 : Constant  Value=10.11
  3 : Constant  Value=10.95
  4 : Constant  Value=11.22
  5 : Constant  Value=10.11
  9 : Constant  Value=10.11
  Abs : Abs
  Add : Sum
  Add1 : Sum  Inputs=++++++
  Add2 : Sum
  Add3 : Sum  Inputs=+++++
  Add4 : Sum  Inputs=++++++
  Compare To Constant1 : simulink/Logic and Bit Operations/Compare To Constant  relop===  const=2  OutDataTypeStr=boolean
  Compare To Constant10 : simulink/Logic and Bit Operations/Compare To Constant  relop===  const=11  OutDataTypeStr=boolean
  Compare To Constant12 : simulink/Logic and Bit Operations/Compare To Constant  relop===  const=1  OutDataTypeStr=boolean
  Compare To Constant13 : simulink/Logic and Bit Operations/Compare To Constant  relop===  const=2  OutDataTypeStr=boolean
  Compare To Constant14 : simulink/Logic and Bit Operations/Compare To Constant  relop===  const=3  OutDataTypeStr=boolean
  Compare To Constant15 : simulink/Logic and Bit Operations/Compare To Constant  relop===  const=4  OutDataTypeStr=boolean
  Compare To Constant16 : simulink/Logic and Bit Operations/Compare To Constant  relop===  const=1  OutDataTypeStr=boolean
  Compare To Constant17 : simulink/Logic and Bit Operations/Compare To Constant  relop===  const=0  OutDataTypeStr=boolean
  Compare To Constant2 : simulink/Logic and Bit Operations/Compare To Constant  relop===  const=3  OutDataTypeStr=boolean
  Compare To Constant3 : simulink/Logic and Bit Operations/Compare To Constant  relop===  const=4  OutDataTypeStr=boolean
  Compare To Constant4 : simulink/Logic and Bit Operations/Compare To Constant  relop===  const=5  OutDataTypeStr=boolean
  Compare To Constant5 : simulink/Logic and Bit Operations/Compare To Constant  relop===  const=6  OutDataTypeStr=boolean
  Compare To Constant6 : simulink/Logic and Bit Operations/Compare To Constant  relop===  const=7  OutDataTypeStr=boolean
  Compare To Constant7 : simulink/Logic and Bit Operations/Compare To Constant  relop===  const=8  OutDataTypeStr=boolean
  Compare To Constant8 : simulink/Logic and Bit Operations/Compare To Constant  relop===  const=9  OutDataTypeStr=boolean
  Compare To Constant9 : simulink/Logic and Bit Operations/Compare To Constant  relop===  const=10  OutDataTypeStr=boolean
  Compare To Zero : simulink/Logic and Bit Operations/Compare To Zero  relop===  OutDataTypeStr=boolean
  Divide : Product  Inputs=*/
  Divide{1..8,10..13,15..18,20..21} (18 alike) : Product  Inputs=**
  Divide14 : Product  Inputs=*//
  Math Function : Math  Operator=square  SaturateOnIntegerOverflow=on
  tag scope: ohms2=global
  wires:
  Divide1/1 -> [ohms2]
  Compare To Constant13/1 -> Divide18/1
  Add2/1 -> Divide1/1
  Add3/1 -> Divide21/1
  [Test_Num] -> Compare To Constant2/1
  Compare To Constant16/1 -> Divide21/2
  14/1 -> Divide18/2
  [Test_Num] -> Compare To Constant1/1
  Add/1 -> Divide1/2
  Divide13/1 -> Add1/6
  Divide20/1 -> Add3/1
  12/1 -> Divide16/2
  Compare To Constant17/1 -> Divide20/1
  [Sub_Test_Num] -> Compare To Constant17/1
  5/1 -> Divide5/2
  [Test_Num] -> Compare To Constant4/1
  Divide18/1 -> Add3/3
  Divide4/1 -> Add4/5
  Divide16/1 -> Add3/5
  Compare To Constant14/1 -> Divide15/1
  [Sub_Test_Num] -> Compare To Constant13/1
  7/1 -> Divide7/2
  [Sub_Test_Num] -> Compare To Constant12/1
  Compare To Constant2/1 -> Divide3/1
  [Test_Num] -> Compare To Constant16/1
  [Rpot] -> Divide/1
  Divide15/1 -> Add3/4
  Math Function/1 -> Divide14/1
  Divide8/1 -> Add4/1
  15/1 -> Divide15/2
  Compare To Constant15/1 -> Divide16/1
  [Sub_Test_Num] -> Compare To Constant14/1
  Compare To Constant9/1 -> Divide12/1
  Compare To Constant5/1 -> Divide6/1
  [Test_Num] -> Compare To Constant10/1
  Add4/1 -> Add2/2
  [Sub_Test_Num] -> Compare To Constant15/1
  Add1/1 -> Add2/1
  [Test_Num] -> Compare To Constant6/1
  Divide17/1 -> Add3/2
  [Test_Num] -> Compare To Constant8/1
  Compare To Constant6/1 -> Divide7/1
  Divide7/1 -> Add1/2
  [Inv_Size] -> Divide14/2
  9/1 -> Divide10/2
  Divide11/1 -> Add1/4
  Divide14/1 -> Divide13/2
  Compare To Constant8/1 -> Divide11/1
  Divide10/1 -> Add1/3
  [Vll_Inv] -> Math Function/1
  11/1 -> Divide12/2
  Compare To Zero/1 -> Divide8/1
  [Test_Num] -> Compare To Constant5/1
  Compare To Constant10/1 -> Divide13/1
  [Test_Num] -> Compare To Constant7/1
  Compare To Constant4/1 -> Divide5/1
  16/1 -> Divide20/2
  3/1 -> Divide3/2
  100/1 -> Divide/2
  13/1 -> Divide17/2
  Compare To Constant7/1 -> Divide10/1
  Divide/1 -> Add/1
  Abs/1 -> Divide14/3
  4/1 -> Divide4/2
  [Test_Num] -> Compare To Constant9/1
  6/1 -> Divide6/2
  [Test_Num] -> Compare To Constant3/1
  Compare To Constant1/1 -> Divide2/1
  [Test_Num] -> Compare To Zero/1
  Compare To Constant3/1 -> Divide4/1
  [PRcus] -> Abs/1
  Divide12/1 -> Add1/5
  Divide21/1 -> Add4/2
  Divide6/1 -> Add1/1
  Divide3/1 -> Add4/4
  Divide5/1 -> Add4/6
  2/1 -> Divide2/2
  10/1 -> Divide11/2
  Divide2/1 -> Add4/3
  Compare To Constant12/1 -> Divide17/1
  [ohms1] -> Divide8/2
  1/1 -> Add/2

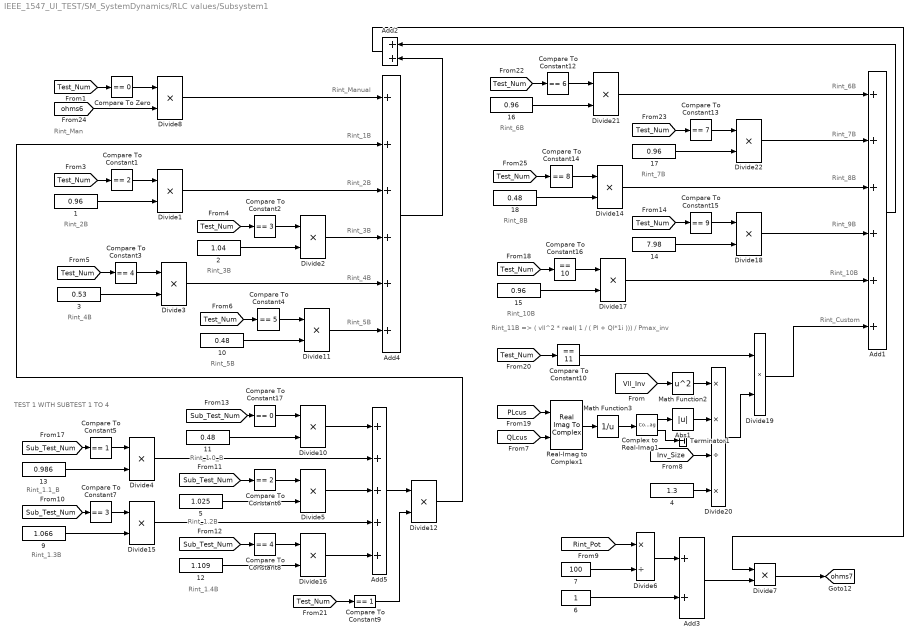
== system IEEE_1547_UI_TEST/SM_SystemDynamics/RLC values/Subsystem1 ==
  note: Rint_Man
  note: Rint_4B
  note: Rint_1B
  note: Rint_11B => ( vll^2 * real( 1 / ( Pl + Ql*1i ))) / Pmax_inv
  note: Rint_1.2B
  note: Rint_8B
  note: Rint_5B
  note: Rint_2B
  note: Rint_3B
  note: Rint_Manual
  note: Rint_1.3B
  note: TEST 1 WITH SUBTEST 1 TO 4
  note: Rint_1.1_B
  note: Rint_9B
  note: Rint_3B
  note: Rint_5B
  note: Rint_10B
  note: Rint_7B
  note: Rint_4B
  note: Rint_1.4B
  note: Rint_Custom
  note: Rint_2B
  note: Rint_10B
  note: Rint_8B
  note: Rint_6B
  note: Rint_7B
  note: Rint_6B
  note: Rint_1.0_B
  {1,15..17} (4 alike) : Constant  Value=0.96
  10 : Constant  Value=0.48
  11 : Constant  Value=0.48
  12 : Constant  Value=1.109
  13 : Constant  Value=0.986
  14 : Constant  Value=7.98
  18 : Constant  Value=0.48
  2 : Constant  Value=1.04
  3 : Constant  Value=0.53
  4 : Constant  Value=1.3
  5 : Constant  Value=1.025
  6 : Constant
  7 : Constant  Value=100
  9 : Constant  Value=1.066
  Abs1 : Abs
  Add1 : Sum  Inputs=++++++
  Add2 : Sum
  Add3 : Sum
  Add4 : Sum  Inputs=++++++
  Add5 : Sum  Inputs=+++++
  Compare To Constant1 : simulink/Logic and Bit Operations/Compare To Constant  relop===  const=2  OutDataTypeStr=boolean
  Compare To Constant10 : simulink/Logic and Bit Operations/Compare To Constant  relop===  const=11  OutDataTypeStr=boolean
  Compare To Constant12 : simulink/Logic and Bit Operations/Compare To Constant  relop===  const=6  OutDataTypeStr=boolean
  Compare To Constant13 : simulink/Logic and Bit Operations/Compare To Constant  relop===  const=7  OutDataTypeStr=boolean
  Compare To Constant14 : simulink/Logic and Bit Operations/Compare To Constant  relop===  const=8  OutDataTypeStr=boolean
  Compare To Constant15 : simulink/Logic and Bit Operations/Compare To Constant  relop===  const=9  OutDataTypeStr=boolean
  Compare To Constant16 : simulink/Logic and Bit Operations/Compare To Constant  relop===  const=10  OutDataTypeStr=boolean
  Compare To Constant17 : simulink/Logic and Bit Operations/Compare To Constant  relop===  const=0  OutDataTypeStr=boolean
  Compare To Constant2 : simulink/Logic and Bit Operations/Compare To Constant  relop===  const=3  OutDataTypeStr=boolean
  Compare To Constant3 : simulink/Logic and Bit Operations/Compare To Constant  relop===  const=4  OutDataTypeStr=boolean
  Compare To Constant4 : simulink/Logic and Bit Operations/Compare To Constant  relop===  const=5  OutDataTypeStr=boolean
  Compare To Constant5 : simulink/Logic and Bit Operations/Compare To Constant  relop===  const=1  OutDataTypeStr=boolean
  Compare To Constant6 : simulink/Logic and Bit Operations/Compare To Constant  relop===  const=2  OutDataTypeStr=boolean
  Compare To Constant7 : simulink/Logic and Bit Operations/Compare To Constant  relop===  const=3  OutDataTypeStr=boolean
  Compare To Constant8 : simulink/Logic and Bit Operations/Compare To Constant  relop===  const=4  OutDataTypeStr=boolean
  Compare To Constant9 : simulink/Logic and Bit Operations/Compare To Constant  relop===  const=1  OutDataTypeStr=boolean
  Compare To Zero : simulink/Logic and Bit Operations/Compare To Zero  relop===  OutDataTypeStr=boolean
  Complex to Real-Imag1 : ComplexToRealImag
  Divide{1..5,7..8,10..12,14..19,21..22} (18 alike) : Product  Inputs=**
  Divide20 : Product  Inputs=**/*
  Divide6 : Product  Inputs=*/
  Math Function2 : Math  Operator=square  SaturateOnIntegerOverflow=on
  Math Function3 : Math  Operator=reciprocal  SaturateOnIntegerOverflow=on
  Real-Imag to Complex1 : RealImagToComplex
  Terminator1 : Terminator
  tag scope: ohms7=global
  wires:
  10/1 -> Divide11/2
  18/1 -> Divide14/2
  Compare To Constant13/1 -> Divide22/1
  Compare To Constant12/1 -> Divide21/1
  16/1 -> Divide21/2
  Compare To Zero/1 -> Divide8/1
  Divide1/1 -> Add4/3
  [Test_Num] -> Compare To Zero/1
  [ohms6] -> Divide8/2
  Compare To Constant3/1 -> Divide3/1
  Compare To Constant16/1 -> Divide17/1
  3/1 -> Divide3/2
  17/1 -> Divide22/2
  Compare To Constant14/1 -> Divide14/1
  Divide12/1 -> Add4/2
  9/1 -> Divide15/2
  Compare To Constant5/1 -> Divide4/1
  Divide10/1 -> Add5/1
  Divide8/1 -> Add4/1
  [Sub_Test_Num] -> Compare To Constant7/1
  Divide14/1 -> Add1/3
  [PLcus] -> Real-Imag to Complex1/1
  Divide22/1 -> Add1/2
  Compare To Constant9/1 -> Divide12/2
  Compare To Constant7/1 -> Divide15/1
  [Sub_Test_Num] -> Compare To Constant8/1
  [Inv_Size] -> Divide20/3
  Divide6/1 -> Add3/1
  [Sub_Test_Num] -> Compare To Constant6/1
  [Test_Num] -> Compare To Constant3/1
  Math Function3/1 -> Complex to Real-Imag1/1
  [Test_Num] -> Compare To Constant14/1
  Compare To Constant8/1 -> Divide16/1
  Divide20/1 -> Divide19/2
  Divide16/1 -> Add5/5
  Add5/1 -> Divide12/1
  12/1 -> Divide16/2
  [QLcus] -> Real-Imag to Complex1/2
  15/1 -> Divide17/2
  Real-Imag to Complex1/1 -> Math Function3/1
  Divide15/1 -> Add5/4
  [Test_Num] -> Compare To Constant9/1
  Compare To Constant17/1 -> Divide10/1
  14/1 -> Divide18/2
  Divide4/1 -> Add5/2
  7/1 -> Divide6/2
  4/1 -> Divide20/4
  Divide5/1 -> Add5/3
  Add1/1 -> Add2/1
  11/1 -> Divide10/2
  Add3/1 -> Divide7/2
  13/1 -> Divide4/2
  [Test_Num] -> Compare To Constant13/1
  Compare To Constant15/1 -> Divide18/1
  Divide21/1 -> Add1/1
  Complex to Real-Imag1/1 -> Abs1/1
  [Sub_Test_Num] -> Compare To Constant5/1
  1/1 -> Divide1/2
  Abs1/1 -> Divide20/2
  Divide17/1 -> Add1/5
  [Rint_Pot] -> Divide6/1
  Add4/1 -> Add2/2
  Divide19/1 -> Add1/6
  [Sub_Test_Num] -> Compare To Constant17/1
  [Vll_Inv] -> Math Function2/1
  Compare To Constant2/1 -> Divide2/1
  [Test_Num] -> Compare To Constant12/1
  Add2/1 -> Divide7/1
  Compare To Constant10/1 -> Divide19/1
  Divide18/1 -> Add1/4
  [Test_Num] -> Compare To Constant15/1
  5/1 -> Divide5/2
  Divide3/1 -> Add4/5
  2/1 -> Divide2/2
  Compare To Constant4/1 -> Divide11/1
  Math Function2/1 -> Divide20/1
  Divide11/1 -> Add4/6
  [Test_Num] -> Compare To Constant4/1
  Divide2/1 -> Add4/4
  Divide7/1 -> [ohms7]
  [Test_Num] -> Compare To Constant10/1
  [Test_Num] -> Compare To Constant1/1
  Compare To Constant1/1 -> Divide1/1
  Complex to Real-Imag1/2 -> Terminator1/1
  [Test_Num] -> Compare To Constant2/1
  Compare To Constant6/1 -> Divide5/1
  6/1 -> Add3/2
  [Test_Num] -> Compare To Constant16/1

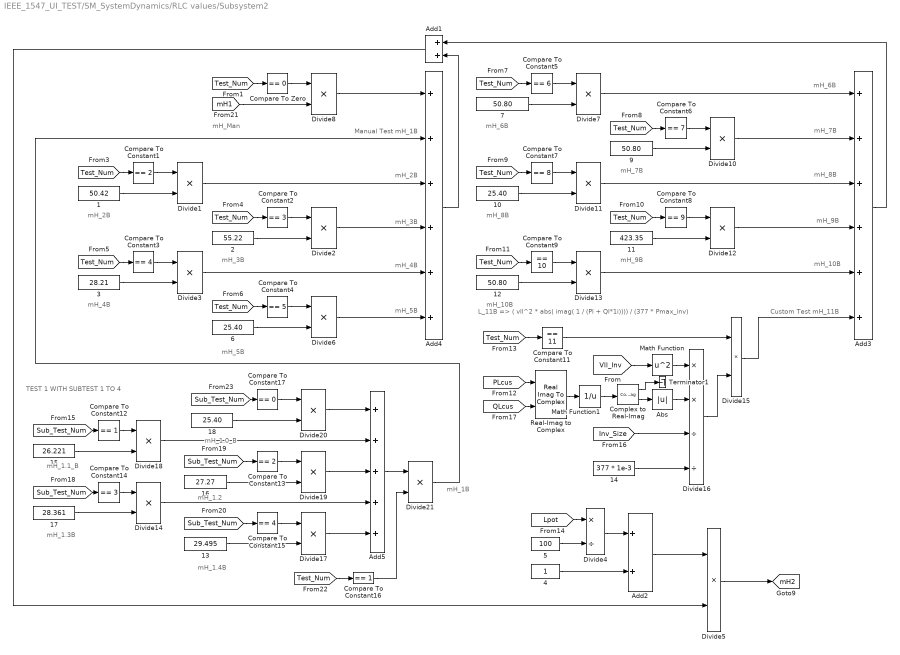
== system IEEE_1547_UI_TEST/SM_SystemDynamics/RLC values/Subsystem2 ==
  note: mH_6B
  note: mH_7B
  note: mH_9B
  note: mH_6B
  note: mH_10B
  note: mH_1.4B
  note: mH_1.2
  note: TEST 1 WITH SUBTEST 1 TO 4
  note: mH_2B
  note: mH_3B
  note: mH_5B
  note: mH_7B
  note: mH_5B
  note: Custom Test mH_11B
  note: mH_10B
  note: mH_1.3B
  note: mH_1.1_B
  note: mH_Man
  note: mH_1B
  note: mH_8B
  note: mH_2B
  note: mH_3B
  note: mH_9B
  note: mH_4B
  note: mH_1.0_B
  note: L_11B => ( vll^2 * abs( imag( 1 / (Pl + Ql*1i)))) / (377 * Pmax_inv)
  note: mH_8B
  note: mH_4B
  note: Manual Test mH_1B
  1 : Constant  Value=50.42
  10 : Constant  Value=25.40
  11 : Constant  Value=423.35
  12 : Constant  Value=50.80
  13 : Constant  Value=29.495
  14 : Constant  Value=377 * 1e-3
  15 : Constant  Value=26.221
  16 : Constant  Value=27.27
  17 : Constant  Value=28.361
  18 : Constant  Value=25.40
  2 : Constant  Value=55.22
  3 : Constant  Value=28.21
  4 : Constant
  5 : Constant  Value=100
  6 : Constant  Value=25.40
  7 : Constant  Value=50.80
  9 : Constant  Value=50.80
  Abs : Abs
  Add1 : Sum
  Add2 : Sum
  Add3 : Sum  Inputs=++++++
  Add4 : Sum  Inputs=++++++
  Add5 : Sum  Inputs=+++++
  Compare To Constant1 : simulink/Logic and Bit Operations/Compare To Constant  relop===  const=2  OutDataTypeStr=boolean
  Compare To Constant11 : simulink/Logic and Bit Operations/Compare To Constant  relop===  const=11  OutDataTypeStr=boolean
  Compare To Constant12 : simulink/Logic and Bit Operations/Compare To Constant  relop===  const=1  OutDataTypeStr=boolean
  Compare To Constant13 : simulink/Logic and Bit Operations/Compare To Constant  relop===  const=2  OutDataTypeStr=boolean
  Compare To Constant14 : simulink/Logic and Bit Operations/Compare To Constant  relop===  const=3  OutDataTypeStr=boolean
  Compare To Constant15 : simulink/Logic and Bit Operations/Compare To Constant  relop===  const=4  OutDataTypeStr=boolean
  Compare To Constant16 : simulink/Logic and Bit Operations/Compare To Constant  relop===  const=1  OutDataTypeStr=boolean
  Compare To Constant17 : simulink/Logic and Bit Operations/Compare To Constant  relop===  const=0  OutDataTypeStr=boolean
  Compare To Constant2 : simulink/Logic and Bit Operations/Compare To Constant  relop===  const=3  OutDataTypeStr=boolean
  Compare To Constant3 : simulink/Logic and Bit Operations/Compare To Constant  relop===  const=4  OutDataTypeStr=boolean
  Compare To Constant4 : simulink/Logic and Bit Operations/Compare To Constant  relop===  const=5  OutDataTypeStr=boolean
  Compare To Constant5 : simulink/Logic and Bit Operations/Compare To Constant  relop===  const=6  OutDataTypeStr=boolean
  Compare To Constant6 : simulink/Logic and Bit Operations/Compare To Constant  relop===  const=7  OutDataTypeStr=boolean
  Compare To Constant7 : simulink/Logic and Bit Operations/Compare To Constant  relop===  const=8  OutDataTypeStr=boolean
  Compare To Constant8 : simulink/Logic and Bit Operations/Compare To Constant  relop===  const=9  OutDataTypeStr=boolean
  Compare To Constant9 : simulink/Logic and Bit Operations/Compare To Constant  relop===  const=10  OutDataTypeStr=boolean
  Compare To Zero : simulink/Logic and Bit Operations/Compare To Zero  relop===  OutDataTypeStr=boolean
  Complex to Real-Imag : ComplexToRealImag
  Divide{1..3,5..8,10..15,17..21} (18 alike) : Product  Inputs=**
  Divide16 : Product  Inputs=**//
  Divide4 : Product  Inputs=*/
  Math Function : Math  Operator=square  SaturateOnIntegerOverflow=on
  Math Function1 : Math  Operator=reciprocal  SaturateOnIntegerOverflow=on
  Real-Imag to Complex : RealImagToComplex
  Terminator1 : Terminator
  tag scope: mH2=global
  wires:
  Divide8/1 -> Add4/1
  [mH1] -> Divide8/2
  Add5/1 -> Divide21/1
  Compare To Zero/1 -> Divide8/1
  [Test_Num] -> Compare To Constant3/1
  Compare To Constant11/1 -> Divide15/1
  10/1 -> Divide11/2
  Add2/1 -> Divide5/1
  [Sub_Test_Num] -> Compare To Constant15/1
  15/1 -> Divide18/2
  [Test_Num] -> Compare To Constant2/1
  Add1/1 -> Divide5/2
  6/1 -> Divide6/2
  Compare To Constant1/1 -> Divide1/1
  Divide10/1 -> Add3/2
  Divide21/1 -> Add4/2
  Compare To Constant14/1 -> Divide14/1
  Compare To Constant17/1 -> Divide20/1
  18/1 -> Divide20/2
  [Sub_Test_Num] -> Compare To Constant13/1
  Compare To Constant15/1 -> Divide17/1
  14/1 -> Divide16/4
  Divide13/1 -> Add3/5
  Divide12/1 -> Add3/4
  [Test_Num] -> Compare To Constant5/1
  Compare To Constant8/1 -> Divide12/1
  Compare To Constant6/1 -> Divide10/1
  [Test_Num] -> Compare To Constant8/1
  Compare To Constant7/1 -> Divide11/1
  [Sub_Test_Num] -> Compare To Constant12/1
  [Lpot] -> Divide4/1
  2/1 -> Divide2/2
  [Test_Num] -> Compare To Constant1/1
  [Test_Num] -> Compare To Constant6/1
  3/1 -> Divide3/2
  [Test_Num] -> Compare To Constant4/1
  Divide4/1 -> Add2/1
  Compare To Constant4/1 -> Divide6/1
  [Inv_Size] -> Divide16/3
  7/1 -> Divide7/2
  1/1 -> Divide1/2
  Compare To Constant3/1 -> Divide3/1
  Compare To Constant9/1 -> Divide13/1
  13/1 -> Divide17/2
  [Test_Num] -> Compare To Constant11/1
  [Sub_Test_Num] -> Compare To Constant14/1
  Compare To Constant16/1 -> Divide21/2
  [Test_Num] -> Compare To Constant7/1
  Divide2/1 -> Add4/4
  Compare To Constant12/1 -> Divide18/1
  [Test_Num] -> Compare To Zero/1
  Compare To Constant13/1 -> Divide19/1
  [QLcus] -> Real-Imag to Complex/2
  Divide19/1 -> Add5/3
  9/1 -> Divide10/2
  11/1 -> Divide12/2
  [Sub_Test_Num] -> Compare To Constant17/1
  5/1 -> Divide4/2
  [Test_Num] -> Compare To Constant16/1
  [PLcus] -> Real-Imag to Complex/1
  17/1 -> Divide14/2
  16/1 -> Divide19/2
  Compare To Constant5/1 -> Divide7/1
  Divide14/1 -> Add5/4
  Divide20/1 -> Add5/1
  [Test_Num] -> Compare To Constant9/1
  Add3/1 -> Add1/1
  [Vll_Inv] -> Math Function/1
  Divide7/1 -> Add3/1
  4/1 -> Add2/2
  Divide6/1 -> Add4/6
  Divide3/1 -> Add4/5
  Complex to Real-Imag/1 -> Terminator1/1
  Abs/1 -> Divide16/2
  Divide11/1 -> Add3/3
  Divide15/1 -> Add3/6
  Divide16/1 -> Divide15/2
  Divide5/1 -> [mH2]
  Divide17/1 -> Add5/5
  Complex to Real-Imag/2 -> Abs/1
  12/1 -> Divide13/2
  Real-Imag to Complex/1 -> Math Function1/1
  Math Function/1 -> Divide16/1
  Compare To Constant2/1 -> Divide2/1
  Math Function1/1 -> Complex to Real-Imag/1
  Add4/1 -> Add1/2
  Divide18/1 -> Add5/2
  Divide1/1 -> Add4/3
